simulink model "Driving_ACC_CACC_TL"  (R2016a)
settings: Solver=VariableStepAuto  StartTime=0.0  StopTime=10.0  RelTol=1e-3
undefined symbols (not defined in the file): ACCDelayDistance, ACCDelayVelocity, Area, ComfortAccelerationParameter, cR, cW, DeltaLeadVelocity, Epsilon, FuelConsumptionFactor, FuelConsumptionOffset, Mass, MaxBreakAcceleration, MaxLeadDistance, MaxSpeed, Power, StandstillDistance, StepTimeCoefficient, TimeGap
(part 1 of 2)
settings Model: Creator=Schlie  LastModifiedBy=Schlie

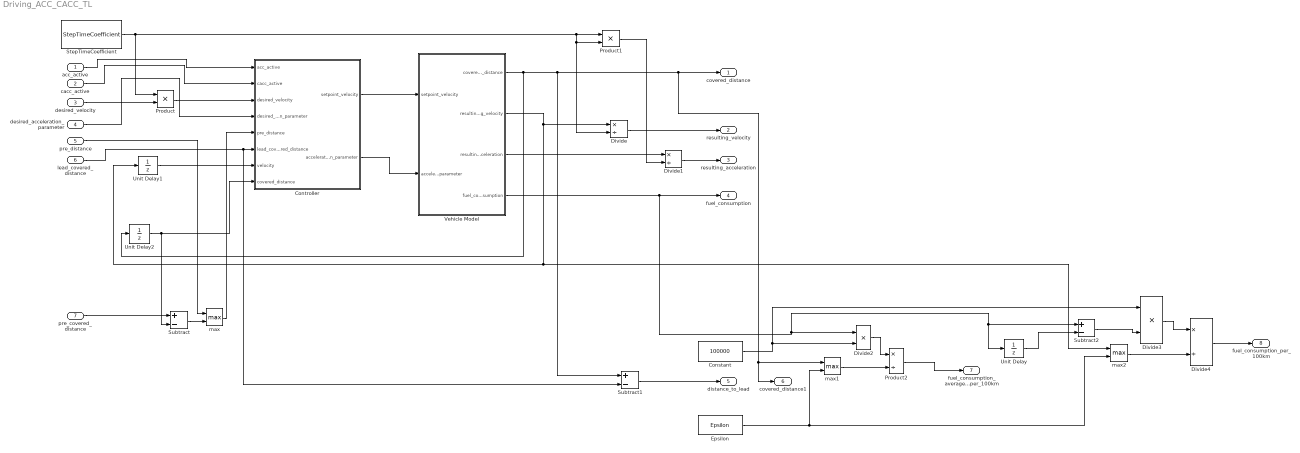
== system Driving_ACC_CACC_TL ==
  acc_active : Inport
      settings: DeleteFcn=if exist('delete_tlblock','file')==2,delete_tlblock(gcbh);end  OpenFcn=if exist('tl_open_blockdlg','file')==2,tl_open_blockdlg(gcbh);else,open_system(gcbh,'parameter');end
      settings: CopyFcn=|
      | if exist('tl_reset_reviewflag','file')==2
      |     tl_reset_reviewflag(gcbh);
      | end
      | if exist('tl_check_ports','file')
      |     tl_check_ports(gcbh);
      | end
      settings: NameChangeFcn=|
      | if exist('rename_tlblock','file')==2,rename_tlblock(gcbh);end
      | if exist('tl_check_ports','file'), tl_check_ports(gcbh); end
  cacc_active : Inport  Port=2
      settings: DeleteFcn=if exist('delete_tlblock','file')==2,delete_tlblock(gcbh);end  OpenFcn=if exist('tl_open_blockdlg','file')==2,tl_open_blockdlg(gcbh);else,open_system(gcbh,'parameter');end
      settings: CopyFcn=|
      | if exist('tl_reset_reviewflag','file')==2
      |     tl_reset_reviewflag(gcbh);
      | end
      | if exist('tl_check_ports','file')
      |     tl_check_ports(gcbh);
      | end
      settings: NameChangeFcn=|
      | if exist('rename_tlblock','file')==2,rename_tlblock(gcbh);end
      | if exist('tl_check_ports','file'), tl_check_ports(gcbh); end
  desired_velocity : Inport  Port=3
      settings: DeleteFcn=if exist('delete_tlblock','file')==2,delete_tlblock(gcbh);end  OpenFcn=if exist('tl_open_blockdlg','file')==2,tl_open_blockdlg(gcbh);else,open_system(gcbh,'parameter');end
      settings: CopyFcn=|
      | if exist('tl_reset_reviewflag','file')==2
      |     tl_reset_reviewflag(gcbh);
      | end
      | if exist('tl_check_ports','file')
      |     tl_check_ports(gcbh);
      | end
      settings: NameChangeFcn=|
      | if exist('rename_tlblock','file')==2,rename_tlblock(gcbh);end
      | if exist('tl_check_ports','file'), tl_check_ports(gcbh); end
  desired_acceleration_parameter : Inport  Port=4
      settings: DeleteFcn=if exist('delete_tlblock','file')==2,delete_tlblock(gcbh);end  OpenFcn=if exist('tl_open_blockdlg','file')==2,tl_open_blockdlg(gcbh);else,open_system(gcbh,'parameter');end
      settings: CopyFcn=|
      | if exist('tl_reset_reviewflag','file')==2
      |     tl_reset_reviewflag(gcbh);
      | end
      | if exist('tl_check_ports','file')
      |     tl_check_ports(gcbh);
      | end
      settings: NameChangeFcn=|
      | if exist('rename_tlblock','file')==2,rename_tlblock(gcbh);end
      | if exist('tl_check_ports','file'), tl_check_ports(gcbh); end
  pre_distance : Inport  Port=5
      settings: DeleteFcn=if exist('delete_tlblock','file')==2,delete_tlblock(gcbh);end  OpenFcn=if exist('tl_open_blockdlg','file')==2,tl_open_blockdlg(gcbh);else,open_system(gcbh,'parameter');end
      settings: CopyFcn=|
      | if exist('tl_reset_reviewflag','file')==2
      |     tl_reset_reviewflag(gcbh);
      | end
      | if exist('tl_check_ports','file')
      |     tl_check_ports(gcbh);
      | end
      settings: NameChangeFcn=|
      | if exist('rename_tlblock','file')==2,rename_tlblock(gcbh);end
      | if exist('tl_check_ports','file'), tl_check_ports(gcbh); end
  lead_covered_distance : Inport  Port=6
      settings: DeleteFcn=if exist('delete_tlblock','file')==2,delete_tlblock(gcbh);end  OpenFcn=if exist('tl_open_blockdlg','file')==2,tl_open_blockdlg(gcbh);else,open_system(gcbh,'parameter');end
      settings: CopyFcn=|
      | if exist('tl_reset_reviewflag','file')==2
      |     tl_reset_reviewflag(gcbh);
      | end
      | if exist('tl_check_ports','file')
      |     tl_check_ports(gcbh);
      | end
      settings: NameChangeFcn=|
      | if exist('rename_tlblock','file')==2,rename_tlblock(gcbh);end
      | if exist('tl_check_ports','file'), tl_check_ports(gcbh); end
  pre_covered_distance : Inport  Port=7
      settings: DeleteFcn=if exist('delete_tlblock','file')==2,delete_tlblock(gcbh);end  OpenFcn=if exist('tl_open_blockdlg','file')==2,tl_open_blockdlg(gcbh);else,open_system(gcbh,'parameter');end
      settings: CopyFcn=|
      | if exist('tl_reset_reviewflag','file')==2
      |     tl_reset_reviewflag(gcbh);
      | end
      | if exist('tl_check_ports','file')
      |     tl_check_ports(gcbh);
      | end
      settings: NameChangeFcn=|
      | if exist('rename_tlblock','file')==2,rename_tlblock(gcbh);end
      | if exist('tl_check_ports','file'), tl_check_ports(gcbh); end
  Constant : Constant  Value=100000
      settings: CopyFcn=if exist('tl_reset_reviewflag','file')==2,tl_reset_reviewflag(gcbh);end  DeleteFcn=if exist('delete_tlblock','file')==2,delete_tlblock(gcbh);end  NameChangeFcn=if exist('rename_tlblock','file')==2,rename_tlblock(gcbh);end  OpenFcn=if exist('tl_open_blockdlg','file')==2,tl_open_blockdlg(gcbh);else,open_system(gcbh,'parameter');end
  Controller : Subsystem
  Divide : Product  Inputs=*/
      settings: CopyFcn=if exist('tl_reset_reviewflag','file')==2,tl_reset_reviewflag(gcbh);end  DeleteFcn=if exist('delete_tlblock','file')==2,delete_tlblock(gcbh);end  NameChangeFcn=if exist('rename_tlblock','file')==2,rename_tlblock(gcbh);end  OpenFcn=if exist('tl_open_blockdlg','file')==2,tl_open_blockdlg(gcbh);else,open_system(gcbh,'parameter');end
  Divide1 : Product  Inputs=*/
      settings: CopyFcn=if exist('tl_reset_reviewflag','file')==2,tl_reset_reviewflag(gcbh);end  DeleteFcn=if exist('delete_tlblock','file')==2,delete_tlblock(gcbh);end  NameChangeFcn=if exist('rename_tlblock','file')==2,rename_tlblock(gcbh);end  OpenFcn=if exist('tl_open_blockdlg','file')==2,tl_open_blockdlg(gcbh);else,open_system(gcbh,'parameter');end
  Divide2 : Product  Inputs=**
      settings: CopyFcn=if exist('tl_reset_reviewflag','file')==2,tl_reset_reviewflag(gcbh);end  DeleteFcn=if exist('delete_tlblock','file')==2,delete_tlblock(gcbh);end  NameChangeFcn=if exist('rename_tlblock','file')==2,rename_tlblock(gcbh);end  OpenFcn=if exist('tl_open_blockdlg','file')==2,tl_open_blockdlg(gcbh);else,open_system(gcbh,'parameter');end
  Divide3 : Product  Inputs=**
      settings: CopyFcn=if exist('tl_reset_reviewflag','file')==2,tl_reset_reviewflag(gcbh);end  DeleteFcn=if exist('delete_tlblock','file')==2,delete_tlblock(gcbh);end  NameChangeFcn=if exist('rename_tlblock','file')==2,rename_tlblock(gcbh);end  OpenFcn=if exist('tl_open_blockdlg','file')==2,tl_open_blockdlg(gcbh);else,open_system(gcbh,'parameter');end
  Divide4 : Product  Inputs=*/
      settings: CopyFcn=if exist('tl_reset_reviewflag','file')==2,tl_reset_reviewflag(gcbh);end  DeleteFcn=if exist('delete_tlblock','file')==2,delete_tlblock(gcbh);end  NameChangeFcn=if exist('rename_tlblock','file')==2,rename_tlblock(gcbh);end  OpenFcn=if exist('tl_open_blockdlg','file')==2,tl_open_blockdlg(gcbh);else,open_system(gcbh,'parameter');end
  Epsilon : Constant  Value=Epsilon
      settings: CopyFcn=if exist('tl_reset_reviewflag','file')==2,tl_reset_reviewflag(gcbh);end  DeleteFcn=if exist('delete_tlblock','file')==2,delete_tlblock(gcbh);end  NameChangeFcn=if exist('rename_tlblock','file')==2,rename_tlblock(gcbh);end  OpenFcn=if exist('tl_open_blockdlg','file')==2,tl_open_blockdlg(gcbh);else,open_system(gcbh,'parameter');end
  Product : Product
      settings: CopyFcn=if exist('tl_reset_reviewflag','file')==2,tl_reset_reviewflag(gcbh);end  DeleteFcn=if exist('delete_tlblock','file')==2,delete_tlblock(gcbh);end  NameChangeFcn=if exist('rename_tlblock','file')==2,rename_tlblock(gcbh);end  OpenFcn=if exist('tl_open_blockdlg','file')==2,tl_open_blockdlg(gcbh);else,open_system(gcbh,'parameter');end
  Product1 : Product
      settings: CopyFcn=if exist('tl_reset_reviewflag','file')==2,tl_reset_reviewflag(gcbh);end  DeleteFcn=if exist('delete_tlblock','file')==2,delete_tlblock(gcbh);end  NameChangeFcn=if exist('rename_tlblock','file')==2,rename_tlblock(gcbh);end  OpenFcn=if exist('tl_open_blockdlg','file')==2,tl_open_blockdlg(gcbh);else,open_system(gcbh,'parameter');end
  Product2 : Product  Inputs=*/  RndMeth=Zero
      settings: CopyFcn=if exist('tl_reset_reviewflag') == 2, tl_reset_reviewflag(gcbh); end; if ~strcmp(get_param(gcbh, 'LinkStatus'), 'implicit') set_param(gcbh,'ReferenceBlock',''); end  DeleteFcn=if exist('delete_tlblock','file')==2,delete_tlblock(gcbh);end  NameChangeFcn=if exist('rename_tlblock','file')==2,rename_tlblock(gcbh);end  OpenFcn=if exist('tl_open_blockdlg','file')==2,tl_open_blockdlg(gcbh);else,open_system(gcbh,'parameter');end
  StepTimeCoefficient : Constant  Value=StepTimeCoefficient
      settings: CopyFcn=if exist('tl_reset_reviewflag','file')==2,tl_reset_reviewflag(gcbh);end  DeleteFcn=if exist('delete_tlblock','file')==2,delete_tlblock(gcbh);end  NameChangeFcn=if exist('rename_tlblock','file')==2,rename_tlblock(gcbh);end  OpenFcn=if exist('tl_open_blockdlg','file')==2,tl_open_blockdlg(gcbh);else,open_system(gcbh,'parameter');end
  Subtract : Sum  Inputs=+-
      settings: CopyFcn=if exist('tl_reset_reviewflag','file')==2,tl_reset_reviewflag(gcbh);end  DeleteFcn=if exist('delete_tlblock','file')==2,delete_tlblock(gcbh);end  NameChangeFcn=if exist('rename_tlblock','file')==2,rename_tlblock(gcbh);end  OpenFcn=if exist('tl_open_blockdlg','file')==2,tl_open_blockdlg(gcbh);else,open_system(gcbh,'parameter');end
  Subtract1 : Sum  Inputs=+-
      settings: CopyFcn=if exist('tl_reset_reviewflag','file')==2,tl_reset_reviewflag(gcbh);end  DeleteFcn=if exist('delete_tlblock','file')==2,delete_tlblock(gcbh);end  NameChangeFcn=if exist('rename_tlblock','file')==2,rename_tlblock(gcbh);end  OpenFcn=if exist('tl_open_blockdlg','file')==2,tl_open_blockdlg(gcbh);else,open_system(gcbh,'parameter');end
  Subtract2 : Sum  Inputs=+-
      settings: CopyFcn=if exist('tl_reset_reviewflag','file')==2,tl_reset_reviewflag(gcbh);end  DeleteFcn=if exist('delete_tlblock','file')==2,delete_tlblock(gcbh);end  NameChangeFcn=if exist('rename_tlblock','file')==2,rename_tlblock(gcbh);end  OpenFcn=if exist('tl_open_blockdlg','file')==2,tl_open_blockdlg(gcbh);else,open_system(gcbh,'parameter');end
  Unit Delay : UnitDelay  SampleTime=-1
      settings: CopyFcn=if exist('tl_reset_reviewflag','file')==2,tl_reset_reviewflag(gcbh);end  DeleteFcn=if exist('delete_tlblock','file')==2,delete_tlblock(gcbh);end  NameChangeFcn=if exist('rename_tlblock','file')==2,rename_tlblock(gcbh);end  OpenFcn=if exist('tl_open_blockdlg','file')==2,tl_open_blockdlg(gcbh);else,open_system(gcbh,'parameter');end
  Unit Delay1 : UnitDelay  SampleTime=-1
      settings: CopyFcn=if exist('tl_reset_reviewflag','file')==2,tl_reset_reviewflag(gcbh);end  DeleteFcn=if exist('delete_tlblock','file')==2,delete_tlblock(gcbh);end  NameChangeFcn=if exist('rename_tlblock','file')==2,rename_tlblock(gcbh);end  OpenFcn=if exist('tl_open_blockdlg','file')==2,tl_open_blockdlg(gcbh);else,open_system(gcbh,'parameter');end
  Unit Delay2 : UnitDelay  SampleTime=-1
      settings: CopyFcn=if exist('tl_reset_reviewflag','file')==2,tl_reset_reviewflag(gcbh);end  DeleteFcn=if exist('delete_tlblock','file')==2,delete_tlblock(gcbh);end  NameChangeFcn=if exist('rename_tlblock','file')==2,rename_tlblock(gcbh);end  OpenFcn=if exist('tl_open_blockdlg','file')==2,tl_open_blockdlg(gcbh);else,open_system(gcbh,'parameter');end
  Vehicle Model : Subsystem
  max : MinMax  Function=max  Inputs=2
      settings: CopyFcn=if exist('tl_reset_reviewflag','file')==2,tl_reset_reviewflag(gcbh);end  DeleteFcn=if exist('delete_tlblock','file')==2,delete_tlblock(gcbh);end  NameChangeFcn=if exist('rename_tlblock','file')==2,rename_tlblock(gcbh);end  OpenFcn=if exist('tl_open_blockdlg','file')==2,tl_open_blockdlg(gcbh);else,open_system(gcbh,'parameter');end
  max1 : MinMax  Function=max  Inputs=2
      settings: CopyFcn=if exist('tl_reset_reviewflag','file')==2,tl_reset_reviewflag(gcbh);end  DeleteFcn=if exist('delete_tlblock','file')==2,delete_tlblock(gcbh);end  NameChangeFcn=if exist('rename_tlblock','file')==2,rename_tlblock(gcbh);end  OpenFcn=if exist('tl_open_blockdlg','file')==2,tl_open_blockdlg(gcbh);else,open_system(gcbh,'parameter');end
  max2 : MinMax  Function=max  Inputs=2
      settings: CopyFcn=if exist('tl_reset_reviewflag','file')==2,tl_reset_reviewflag(gcbh);end  DeleteFcn=if exist('delete_tlblock','file')==2,delete_tlblock(gcbh);end  NameChangeFcn=if exist('rename_tlblock','file')==2,rename_tlblock(gcbh);end  OpenFcn=if exist('tl_open_blockdlg','file')==2,tl_open_blockdlg(gcbh);else,open_system(gcbh,'parameter');end
  covered_distance : Outport
      settings: DeleteFcn=if exist('delete_tlblock','file')==2,delete_tlblock(gcbh);end  OpenFcn=if exist('tl_open_blockdlg','file')==2,tl_open_blockdlg(gcbh);else,open_system(gcbh,'parameter');end
      settings: CopyFcn=|
      | if exist('tl_reset_reviewflag','file')==2
      |     tl_reset_reviewflag(gcbh);
      | end
      | if exist('tl_check_ports','file')
      |     tl_check_ports(gcbh);
      | end
      settings: NameChangeFcn=|
      | if exist('rename_tlblock','file')==2,rename_tlblock(gcbh);end
      | if exist('tl_check_ports','file'), tl_check_ports(gcbh); end
  resulting_velocity : Outport  Port=2
      settings: DeleteFcn=if exist('delete_tlblock','file')==2,delete_tlblock(gcbh);end  OpenFcn=if exist('tl_open_blockdlg','file')==2,tl_open_blockdlg(gcbh);else,open_system(gcbh,'parameter');end
      settings: CopyFcn=|
      | if exist('tl_reset_reviewflag','file')==2
      |     tl_reset_reviewflag(gcbh);
      | end
      | if exist('tl_check_ports','file')
      |     tl_check_ports(gcbh);
      | end
      settings: NameChangeFcn=|
      | if exist('rename_tlblock','file')==2,rename_tlblock(gcbh);end
      | if exist('tl_check_ports','file'), tl_check_ports(gcbh); end
  resulting_acceleration : Outport  Port=3
      settings: DeleteFcn=if exist('delete_tlblock','file')==2,delete_tlblock(gcbh);end  OpenFcn=if exist('tl_open_blockdlg','file')==2,tl_open_blockdlg(gcbh);else,open_system(gcbh,'parameter');end
      settings: CopyFcn=|
      | if exist('tl_reset_reviewflag','file')==2
      |     tl_reset_reviewflag(gcbh);
      | end
      | if exist('tl_check_ports','file')
      |     tl_check_ports(gcbh);
      | end
      settings: NameChangeFcn=|
      | if exist('rename_tlblock','file')==2,rename_tlblock(gcbh);end
      | if exist('tl_check_ports','file'), tl_check_ports(gcbh); end
  fuel_consumption : Outport  Port=4
      settings: DeleteFcn=if exist('delete_tlblock','file')==2,delete_tlblock(gcbh);end  OpenFcn=if exist('tl_open_blockdlg','file')==2,tl_open_blockdlg(gcbh);else,open_system(gcbh,'parameter');end
      settings: CopyFcn=|
      | if exist('tl_reset_reviewflag','file')==2
      |     tl_reset_reviewflag(gcbh);
      | end
      | if exist('tl_check_ports','file')
      |     tl_check_ports(gcbh);
      | end
      settings: NameChangeFcn=|
      | if exist('rename_tlblock','file')==2,rename_tlblock(gcbh);end
      | if exist('tl_check_ports','file'), tl_check_ports(gcbh); end
  distance_to_lead : Outport  Port=5
      settings: DeleteFcn=if exist('delete_tlblock','file')==2,delete_tlblock(gcbh);end  OpenFcn=if exist('tl_open_blockdlg','file')==2,tl_open_blockdlg(gcbh);else,open_system(gcbh,'parameter');end
      settings: CopyFcn=|
      | if exist('tl_reset_reviewflag','file')==2
      |     tl_reset_reviewflag(gcbh);
      | end
      | if exist('tl_check_ports','file')
      |     tl_check_ports(gcbh);
      | end
      settings: NameChangeFcn=|
      | if exist('rename_tlblock','file')==2,rename_tlblock(gcbh);end
      | if exist('tl_check_ports','file'), tl_check_ports(gcbh); end
  covered_distance1 : Outport  Port=6
      settings: DeleteFcn=if exist('delete_tlblock','file')==2,delete_tlblock(gcbh);end  OpenFcn=if exist('tl_open_blockdlg','file')==2,tl_open_blockdlg(gcbh);else,open_system(gcbh,'parameter');end
      settings: CopyFcn=|
      | if exist('tl_reset_reviewflag','file')==2
      |     tl_reset_reviewflag(gcbh);
      | end
      | if exist('tl_check_ports','file')
      |     tl_check_ports(gcbh);
      | end
      settings: NameChangeFcn=|
      | if exist('rename_tlblock','file')==2,rename_tlblock(gcbh);end
      | if exist('tl_check_ports','file'), tl_check_ports(gcbh); end
  fuel_consumption_average_per_100km : Outport  Port=7
      settings: DeleteFcn=if exist('delete_tlblock','file')==2,delete_tlblock(gcbh);end  OpenFcn=if exist('tl_open_blockdlg','file')==2,tl_open_blockdlg(gcbh);else,open_system(gcbh,'parameter');end
      settings: CopyFcn=|
      | if exist('tl_reset_reviewflag','file')==2
      |     tl_reset_reviewflag(gcbh);
      | end
      | if exist('tl_check_ports','file')
      |     tl_check_ports(gcbh);
      | end
      settings: NameChangeFcn=|
      | if exist('rename_tlblock','file')==2,rename_tlblock(gcbh);end
      | if exist('tl_check_ports','file'), tl_check_ports(gcbh); end
  fuel_consumption_per_100km : Outport  Port=8
      settings: DeleteFcn=if exist('delete_tlblock','file')==2,delete_tlblock(gcbh);end  OpenFcn=if exist('tl_open_blockdlg','file')==2,tl_open_blockdlg(gcbh);else,open_system(gcbh,'parameter');end
      settings: CopyFcn=|
      | if exist('tl_reset_reviewflag','file')==2
      |     tl_reset_reviewflag(gcbh);
      | end
      | if exist('tl_check_ports','file')
      |     tl_check_ports(gcbh);
      | end
      settings: NameChangeFcn=|
      | if exist('rename_tlblock','file')==2,rename_tlblock(gcbh);end
      | if exist('tl_check_ports','file'), tl_check_ports(gcbh); end
  wires:
  lead_covered_distance/1 -> Subtract1/2, Controller/6(lead_covered_distance)
  Vehicle Model/2(resulting_velocity) -> Divide/1, Unit Delay1/1, max2/1
  acc_active/1 -> Controller/1(acc_active)
  desired_velocity/1 -> Product/2
  StepTimeCoefficient/1 -> Product1/1, Product1/2, Divide/2, Product/1
  Divide1/1 -> resulting_acceleration/1
  Vehicle Model/1(covered_distance) -> Unit Delay2/1, Subtract1/1, covered_distance/1, covered_distance1/1, max1/1
  Divide/1 -> resulting_velocity/1
  cacc_active/1 -> Controller/2(cacc_active)
  Product/1 -> Controller/3(desired_velocity)
  pre_distance/1 -> max/1
  Vehicle Model/3(resulting_acceleration) -> Divide1/1
  Controller/2(acceleration_parameter) -> Vehicle Model/2(acceleration_parameter)
  Constant/1 -> Divide3/1, Divide2/2
  Controller/1(setpoint_velocity) -> Vehicle Model/1(setpoint_velocity)
  Subtract2/1 -> Divide3/2
  max1/1 -> Product2/2
  Subtract/1 -> max/2
  Unit Delay/1 -> Subtract2/2
  pre_covered_distance/1 -> Subtract/1
  Subtract1/1 -> distance_to_lead/1
  Vehicle Model/4(fuel_consumption) -> fuel_consumption/1, Unit Delay/1, Subtract2/1, Divide2/1
  max2/1 -> Divide4/2
  desired_acceleration_parameter/1 -> Controller/4(desired_acceleration_parameter)
  Epsilon/1 -> max2/2, max1/2
  max/1 -> Controller/5(pre_distance)
  Product1/1 -> Divide1/2
  Unit Delay1/1 -> Controller/7(velocity)
  Unit Delay2/1 -> Controller/8(covered_distance), Subtract/2
  Divide2/1 -> Product2/1
  Product2/1 -> fuel_consumption_average_per_100km/1
  Divide3/1 -> Divide4/1
  Divide4/1 -> fuel_consumption_per_100km/1

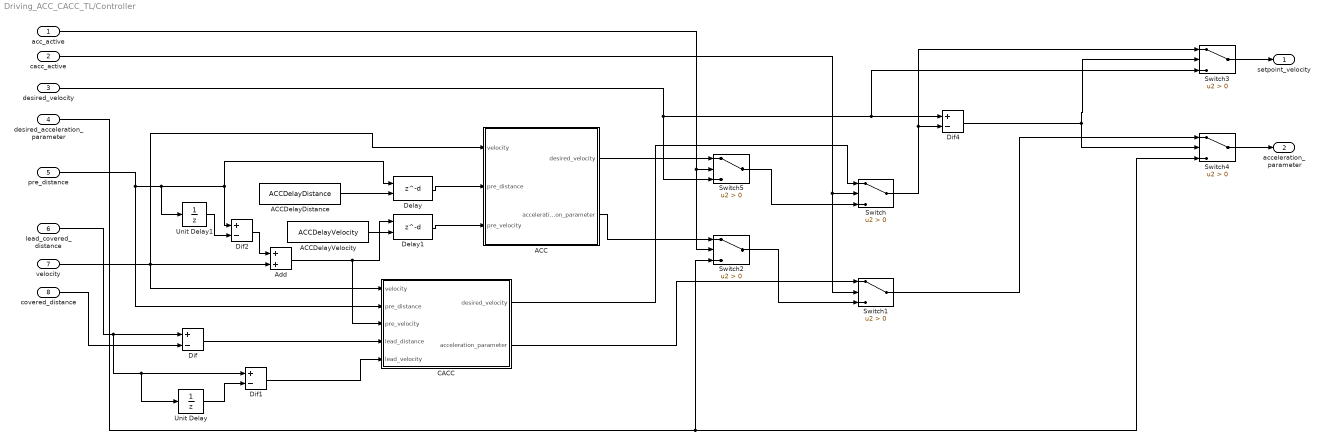
== system Driving_ACC_CACC_TL/Controller ==
  acc_active : Inport
      settings: CopyFcn=if exist('tl_reset_reviewflag','file')==2,tl_reset_reviewflag(gcbh);end  DeleteFcn=if exist('delete_tlblock','file')==2,delete_tlblock(gcbh);end  NameChangeFcn=if exist('rename_tlblock','file')==2,rename_tlblock(gcbh);end  OpenFcn=if exist('tl_open_blockdlg','file')==2,tl_open_blockdlg(gcbh);else,open_system(gcbh,'parameter');end
  cacc_active : Inport  Port=2
      settings: CopyFcn=if exist('tl_reset_reviewflag','file')==2,tl_reset_reviewflag(gcbh);end  DeleteFcn=if exist('delete_tlblock','file')==2,delete_tlblock(gcbh);end  NameChangeFcn=if exist('rename_tlblock','file')==2,rename_tlblock(gcbh);end  OpenFcn=if exist('tl_open_blockdlg','file')==2,tl_open_blockdlg(gcbh);else,open_system(gcbh,'parameter');end
  desired_velocity : Inport  Port=3
      settings: CopyFcn=if exist('tl_reset_reviewflag','file')==2,tl_reset_reviewflag(gcbh);end  DeleteFcn=if exist('delete_tlblock','file')==2,delete_tlblock(gcbh);end  NameChangeFcn=if exist('rename_tlblock','file')==2,rename_tlblock(gcbh);end  OpenFcn=if exist('tl_open_blockdlg','file')==2,tl_open_blockdlg(gcbh);else,open_system(gcbh,'parameter');end
  desired_acceleration_parameter : Inport  Port=4
      settings: CopyFcn=if exist('tl_reset_reviewflag','file')==2,tl_reset_reviewflag(gcbh);end  DeleteFcn=if exist('delete_tlblock','file')==2,delete_tlblock(gcbh);end  NameChangeFcn=if exist('rename_tlblock','file')==2,rename_tlblock(gcbh);end  OpenFcn=if exist('tl_open_blockdlg','file')==2,tl_open_blockdlg(gcbh);else,open_system(gcbh,'parameter');end
  pre_distance : Inport  Port=5
      settings: CopyFcn=if exist('tl_reset_reviewflag','file')==2,tl_reset_reviewflag(gcbh);end  DeleteFcn=if exist('delete_tlblock','file')==2,delete_tlblock(gcbh);end  NameChangeFcn=if exist('rename_tlblock','file')==2,rename_tlblock(gcbh);end  OpenFcn=if exist('tl_open_blockdlg','file')==2,tl_open_blockdlg(gcbh);else,open_system(gcbh,'parameter');end
  lead_covered_distance : Inport  Port=6
      settings: CopyFcn=if exist('tl_reset_reviewflag','file')==2,tl_reset_reviewflag(gcbh);end  DeleteFcn=if exist('delete_tlblock','file')==2,delete_tlblock(gcbh);end  NameChangeFcn=if exist('rename_tlblock','file')==2,rename_tlblock(gcbh);end  OpenFcn=if exist('tl_open_blockdlg','file')==2,tl_open_blockdlg(gcbh);else,open_system(gcbh,'parameter');end
  velocity : Inport  Port=7
      settings: CopyFcn=if exist('tl_reset_reviewflag','file')==2,tl_reset_reviewflag(gcbh);end  DeleteFcn=if exist('delete_tlblock','file')==2,delete_tlblock(gcbh);end  NameChangeFcn=if exist('rename_tlblock','file')==2,rename_tlblock(gcbh);end  OpenFcn=if exist('tl_open_blockdlg','file')==2,tl_open_blockdlg(gcbh);else,open_system(gcbh,'parameter');end
  covered_distance : Inport  Port=8
      settings: CopyFcn=if exist('tl_reset_reviewflag','file')==2,tl_reset_reviewflag(gcbh);end  DeleteFcn=if exist('delete_tlblock','file')==2,delete_tlblock(gcbh);end  NameChangeFcn=if exist('rename_tlblock','file')==2,rename_tlblock(gcbh);end  OpenFcn=if exist('tl_open_blockdlg','file')==2,tl_open_blockdlg(gcbh);else,open_system(gcbh,'parameter');end
  ACC : Subsystem
  ACCDelayDistance : Constant  Value=ACCDelayDistance
      settings: CopyFcn=if exist('tl_reset_reviewflag','file')==2,tl_reset_reviewflag(gcbh);end  DeleteFcn=if exist('delete_tlblock','file')==2,delete_tlblock(gcbh);end  NameChangeFcn=if exist('rename_tlblock','file')==2,rename_tlblock(gcbh);end  OpenFcn=if exist('tl_open_blockdlg','file')==2,tl_open_blockdlg(gcbh);else,open_system(gcbh,'parameter');end
  ACCDelayVelocity : Constant  Value=ACCDelayVelocity
      settings: CopyFcn=if exist('tl_reset_reviewflag','file')==2,tl_reset_reviewflag(gcbh);end  DeleteFcn=if exist('delete_tlblock','file')==2,delete_tlblock(gcbh);end  NameChangeFcn=if exist('rename_tlblock','file')==2,rename_tlblock(gcbh);end  OpenFcn=if exist('tl_open_blockdlg','file')==2,tl_open_blockdlg(gcbh);else,open_system(gcbh,'parameter');end
  Add : Sum
      settings: CopyFcn=if exist('tl_reset_reviewflag','file')==2,tl_reset_reviewflag(gcbh);end  DeleteFcn=if exist('delete_tlblock','file')==2,delete_tlblock(gcbh);end  NameChangeFcn=if exist('rename_tlblock','file')==2,rename_tlblock(gcbh);end  OpenFcn=if exist('tl_open_blockdlg','file')==2,tl_open_blockdlg(gcbh);else,open_system(gcbh,'parameter');end
  CACC : Subsystem
  Delay : Delay  DelayLengthSource=Input port  DelayLength=ACCDelayDistance
      settings: CopyFcn=if exist('tl_reset_reviewflag','file')==2,tl_reset_reviewflag(gcbh);end  DeleteFcn=if exist('delete_tlblock','file')==2,delete_tlblock(gcbh);end  NameChangeFcn=if exist('rename_tlblock','file')==2,rename_tlblock(gcbh);end  OpenFcn=if exist('tl_open_blockdlg','file')==2,tl_open_blockdlg(gcbh);else,open_system(gcbh,'parameter');end  InputPortMap=u0,p1
  Delay1 : Delay  DelayLengthSource=Input port  DelayLength=ACCDelayVelocity
      settings: CopyFcn=if exist('tl_reset_reviewflag','file')==2,tl_reset_reviewflag(gcbh);end  DeleteFcn=if exist('delete_tlblock','file')==2,delete_tlblock(gcbh);end  NameChangeFcn=if exist('rename_tlblock','file')==2,rename_tlblock(gcbh);end  OpenFcn=if exist('tl_open_blockdlg','file')==2,tl_open_blockdlg(gcbh);else,open_system(gcbh,'parameter');end  InputPortMap=u0,p1
  Dif{,1..2,4} (4 alike) : Sum  Inputs=+-
      settings: CopyFcn=if exist('tl_reset_reviewflag','file')==2,tl_reset_reviewflag(gcbh);end  DeleteFcn=if exist('delete_tlblock','file')==2,delete_tlblock(gcbh);end  NameChangeFcn=if exist('rename_tlblock','file')==2,rename_tlblock(gcbh);end  OpenFcn=if exist('tl_open_blockdlg','file')==2,tl_open_blockdlg(gcbh);else,open_system(gcbh,'parameter');end
  Switch{,1..5} (6 alike) : Switch  Criteria=u2 > Threshold
      settings: CopyFcn=if exist('tl_reset_reviewflag','file')==2,tl_reset_reviewflag(gcbh);end  DeleteFcn=if exist('delete_tlblock','file')==2,delete_tlblock(gcbh);end  NameChangeFcn=if exist('rename_tlblock','file')==2,rename_tlblock(gcbh);end  OpenFcn=if exist('tl_open_blockdlg','file')==2,tl_open_blockdlg(gcbh);else,open_system(gcbh,'parameter');end
  Unit Delay : UnitDelay  SampleTime=-1
      settings: CopyFcn=if exist('tl_reset_reviewflag','file')==2,tl_reset_reviewflag(gcbh);end  DeleteFcn=if exist('delete_tlblock','file')==2,delete_tlblock(gcbh);end  NameChangeFcn=if exist('rename_tlblock','file')==2,rename_tlblock(gcbh);end  OpenFcn=if exist('tl_open_blockdlg','file')==2,tl_open_blockdlg(gcbh);else,open_system(gcbh,'parameter');end
  Unit Delay1 : UnitDelay  SampleTime=-1
      settings: CopyFcn=if exist('tl_reset_reviewflag','file')==2,tl_reset_reviewflag(gcbh);end  DeleteFcn=if exist('delete_tlblock','file')==2,delete_tlblock(gcbh);end  NameChangeFcn=if exist('rename_tlblock','file')==2,rename_tlblock(gcbh);end  OpenFcn=if exist('tl_open_blockdlg','file')==2,tl_open_blockdlg(gcbh);else,open_system(gcbh,'parameter');end
  setpoint_velocity : Outport
      settings: CopyFcn=if exist('tl_reset_reviewflag','file')==2,tl_reset_reviewflag(gcbh);end  DeleteFcn=if exist('delete_tlblock','file')==2,delete_tlblock(gcbh);end  NameChangeFcn=if exist('rename_tlblock','file')==2,rename_tlblock(gcbh);end  OpenFcn=if exist('tl_open_blockdlg','file')==2,tl_open_blockdlg(gcbh);else,open_system(gcbh,'parameter');end
  acceleration_parameter : Outport  Port=2
      settings: CopyFcn=if exist('tl_reset_reviewflag','file')==2,tl_reset_reviewflag(gcbh);end  DeleteFcn=if exist('delete_tlblock','file')==2,delete_tlblock(gcbh);end  NameChangeFcn=if exist('rename_tlblock','file')==2,rename_tlblock(gcbh);end  OpenFcn=if exist('tl_open_blockdlg','file')==2,tl_open_blockdlg(gcbh);else,open_system(gcbh,'parameter');end
  wires:
  velocity/1 -> ACC/1(velocity), Add/2, CACC/1(velocity)
  Add/1 -> Delay1/1, CACC/3(pre_velocity)
  lead_covered_distance/1 -> Unit Delay/1, Dif1/1, Dif/1
  covered_distance/1 -> Dif/2
  Dif/1 -> CACC/4(lead_distance)
  Dif1/1 -> CACC/5(lead_velocity)
  Switch3/1 -> setpoint_velocity/1
  desired_velocity/1 -> Switch5/3, Switch3/3, Dif4/1
  Switch4/1 -> acceleration_parameter/1
  Dif2/1 -> Add/1
  Unit Delay/1 -> Dif1/2
  pre_distance/1 -> CACC/2(pre_distance), Unit Delay1/1, Delay/1, Dif2/1
  desired_acceleration_parameter/1 -> Switch2/3, Switch4/3
  Delay/1 -> ACC/2(pre_distance)
  Delay1/1 -> ACC/3(pre_velocity)
  Switch/1 -> Switch3/1, Dif4/2
  Dif4/1 -> Switch3/2, Switch4/2
  Switch1/1 -> Switch4/1
  cacc_active/1 -> Switch1/2, Switch/2
  CACC/1(desired_velocity) -> Switch/1
  CACC/2(acceleration_parameter) -> Switch1/1
  Switch2/1 -> Switch1/3
  Switch5/1 -> Switch/3
  acc_active/1 -> Switch2/2, Switch5/2
  ACC/2(acceleration_parameter) -> Switch2/1
  ACC/1(desired_velocity) -> Switch5/1
  ACCDelayDistance/1 -> Delay/2
  ACCDelayVelocity/1 -> Delay1/2
  Unit Delay1/1 -> Dif2/2

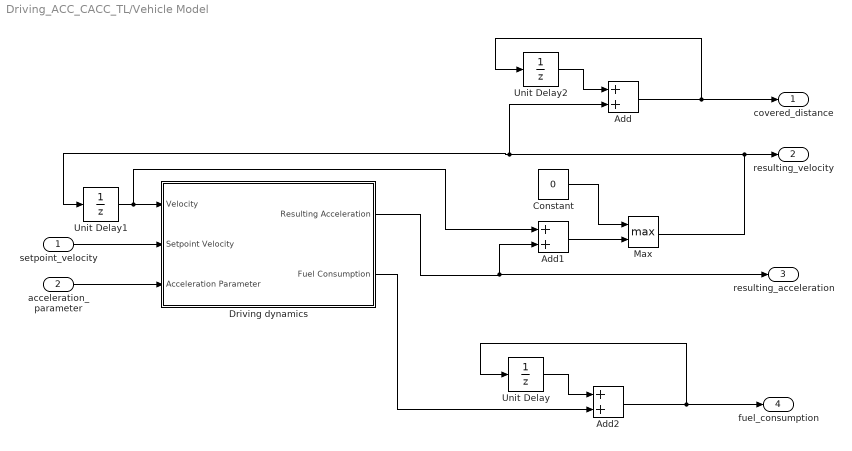
== system Driving_ACC_CACC_TL/Vehicle Model ==
  setpoint_velocity : Inport
  acceleration_parameter : Inport  Port=2
  Add : Sum
      settings: CopyFcn=if exist('tl_reset_reviewflag','file')==2,tl_reset_reviewflag(gcbh);end  DeleteFcn=if exist('delete_tlblock','file')==2,delete_tlblock(gcbh);end  NameChangeFcn=if exist('rename_tlblock','file')==2,rename_tlblock(gcbh);end  OpenFcn=if exist('tl_open_blockdlg','file')==2,tl_open_blockdlg(gcbh);else,open_system(gcbh,'parameter');end
  Add1 : Sum
      settings: CopyFcn=if exist('tl_reset_reviewflag','file')==2,tl_reset_reviewflag(gcbh);end  DeleteFcn=if exist('delete_tlblock','file')==2,delete_tlblock(gcbh);end  NameChangeFcn=if exist('rename_tlblock','file')==2,rename_tlblock(gcbh);end  OpenFcn=if exist('tl_open_blockdlg','file')==2,tl_open_blockdlg(gcbh);else,open_system(gcbh,'parameter');end
  Add2 : Sum
      settings: CopyFcn=if exist('tl_reset_reviewflag','file')==2,tl_reset_reviewflag(gcbh);end  DeleteFcn=if exist('delete_tlblock','file')==2,delete_tlblock(gcbh);end  NameChangeFcn=if exist('rename_tlblock','file')==2,rename_tlblock(gcbh);end  OpenFcn=if exist('tl_open_blockdlg','file')==2,tl_open_blockdlg(gcbh);else,open_system(gcbh,'parameter');end
  Constant : Constant  Value=0
      settings: CopyFcn=if exist('tl_reset_reviewflag','file')==2,tl_reset_reviewflag(gcbh);end  DeleteFcn=if exist('delete_tlblock','file')==2,delete_tlblock(gcbh);end  NameChangeFcn=if exist('rename_tlblock','file')==2,rename_tlblock(gcbh);end  OpenFcn=if exist('tl_open_blockdlg','file')==2,tl_open_blockdlg(gcbh);else,open_system(gcbh,'parameter');end
  Driving dynamics : Subsystem
  Max : MinMax  Function=max  Inputs=2
      settings: CopyFcn=if exist('tl_reset_reviewflag','file')==2,tl_reset_reviewflag(gcbh);end  DeleteFcn=if exist('delete_tlblock','file')==2,delete_tlblock(gcbh);end  NameChangeFcn=if exist('rename_tlblock','file')==2,rename_tlblock(gcbh);end  OpenFcn=if exist('tl_open_blockdlg','file')==2,tl_open_blockdlg(gcbh);else,open_system(gcbh,'parameter');end
  Unit Delay : UnitDelay  SampleTime=-1
      settings: CopyFcn=if exist('tl_reset_reviewflag','file')==2,tl_reset_reviewflag(gcbh);end  DeleteFcn=if exist('delete_tlblock','file')==2,delete_tlblock(gcbh);end  NameChangeFcn=if exist('rename_tlblock','file')==2,rename_tlblock(gcbh);end  OpenFcn=if exist('tl_open_blockdlg','file')==2,tl_open_blockdlg(gcbh);else,open_system(gcbh,'parameter');end
  Unit Delay1 : UnitDelay  SampleTime=-1
      settings: CopyFcn=if exist('tl_reset_reviewflag','file')==2,tl_reset_reviewflag(gcbh);end  DeleteFcn=if exist('delete_tlblock','file')==2,delete_tlblock(gcbh);end  NameChangeFcn=if exist('rename_tlblock','file')==2,rename_tlblock(gcbh);end  OpenFcn=if exist('tl_open_blockdlg','file')==2,tl_open_blockdlg(gcbh);else,open_system(gcbh,'parameter');end
  Unit Delay2 : UnitDelay  SampleTime=-1
      settings: CopyFcn=if exist('tl_reset_reviewflag','file')==2,tl_reset_reviewflag(gcbh);end  DeleteFcn=if exist('delete_tlblock','file')==2,delete_tlblock(gcbh);end  NameChangeFcn=if exist('rename_tlblock','file')==2,rename_tlblock(gcbh);end  OpenFcn=if exist('tl_open_blockdlg','file')==2,tl_open_blockdlg(gcbh);else,open_system(gcbh,'parameter');end
  covered_distance : Outport
  resulting_velocity : Outport  Port=2
  resulting_acceleration : Outport  Port=3
  fuel_consumption : Outport  Port=4
  wires:
  Add/1 -> Unit Delay2/1, covered_distance/1
  Max/1 -> Unit Delay1/1, Add/2, resulting_velocity/1
  setpoint_velocity/1 -> Driving dynamics/2(Setpoint Velocity)
  acceleration_parameter/1 -> Driving dynamics/3(Acceleration Parameter)
  Unit Delay1/1 -> Add1/1, Driving dynamics/1(Velocity)
  Unit Delay2/1 -> Add/1
  Driving dynamics/1(Resulting Acceleration) -> Add1/2, resulting_acceleration/1
  Add1/1 -> Max/2
  Constant/1 -> Max/1
  Add2/1 -> Unit Delay/1, fuel_consumption/1
  Driving dynamics/2(Fuel Consumption) -> Add2/2
  Unit Delay/1 -> Add2/1

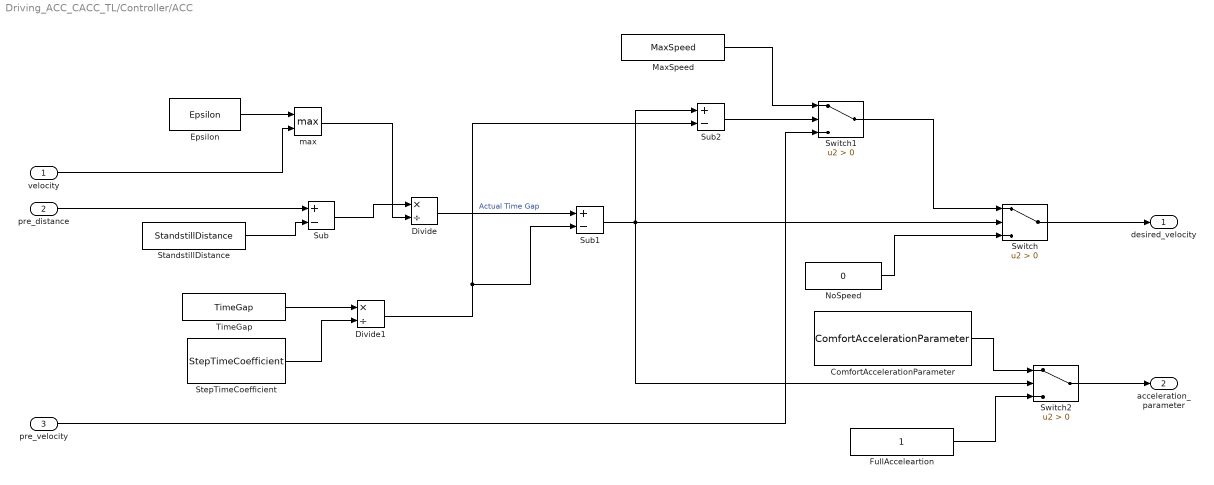
== system Driving_ACC_CACC_TL/Controller/ACC ==
  velocity : Inport
  pre_distance : Inport  Port=2
  pre_velocity : Inport  Port=3
  ComfortAccelerationParameter : Constant  Value=ComfortAccelerationParameter
      settings: CopyFcn=if exist('tl_reset_reviewflag','file')==2,tl_reset_reviewflag(gcbh);end  DeleteFcn=if exist('delete_tlblock','file')==2,delete_tlblock(gcbh);end  NameChangeFcn=if exist('rename_tlblock','file')==2,rename_tlblock(gcbh);end  OpenFcn=if exist('tl_open_blockdlg','file')==2,tl_open_blockdlg(gcbh);else,open_system(gcbh,'parameter');end
  Divide : Product  Inputs=*/
      settings: CopyFcn=if exist('tl_reset_reviewflag','file')==2,tl_reset_reviewflag(gcbh);end  DeleteFcn=if exist('delete_tlblock','file')==2,delete_tlblock(gcbh);end  NameChangeFcn=if exist('rename_tlblock','file')==2,rename_tlblock(gcbh);end  OpenFcn=if exist('tl_open_blockdlg','file')==2,tl_open_blockdlg(gcbh);else,open_system(gcbh,'parameter');end
  Divide1 : Product  Inputs=*/
      settings: CopyFcn=if exist('tl_reset_reviewflag','file')==2,tl_reset_reviewflag(gcbh);end  DeleteFcn=if exist('delete_tlblock','file')==2,delete_tlblock(gcbh);end  NameChangeFcn=if exist('rename_tlblock','file')==2,rename_tlblock(gcbh);end  OpenFcn=if exist('tl_open_blockdlg','file')==2,tl_open_blockdlg(gcbh);else,open_system(gcbh,'parameter');end
  Epsilon : Constant  Value=Epsilon
      settings: CopyFcn=if exist('tl_reset_reviewflag','file')==2,tl_reset_reviewflag(gcbh);end  DeleteFcn=if exist('delete_tlblock','file')==2,delete_tlblock(gcbh);end  NameChangeFcn=if exist('rename_tlblock','file')==2,rename_tlblock(gcbh);end  OpenFcn=if exist('tl_open_blockdlg','file')==2,tl_open_blockdlg(gcbh);else,open_system(gcbh,'parameter');end
  FullAcceleartion : Constant
      settings: CopyFcn=if exist('tl_reset_reviewflag','file')==2,tl_reset_reviewflag(gcbh);end  DeleteFcn=if exist('delete_tlblock','file')==2,delete_tlblock(gcbh);end  NameChangeFcn=if exist('rename_tlblock','file')==2,rename_tlblock(gcbh);end  OpenFcn=if exist('tl_open_blockdlg','file')==2,tl_open_blockdlg(gcbh);else,open_system(gcbh,'parameter');end
  MaxSpeed : Constant  Value=MaxSpeed
      settings: CopyFcn=if exist('tl_reset_reviewflag','file')==2,tl_reset_reviewflag(gcbh);end  DeleteFcn=if exist('delete_tlblock','file')==2,delete_tlblock(gcbh);end  NameChangeFcn=if exist('rename_tlblock','file')==2,rename_tlblock(gcbh);end  OpenFcn=if exist('tl_open_blockdlg','file')==2,tl_open_blockdlg(gcbh);else,open_system(gcbh,'parameter');end
  NoSpeed : Constant  Value=0
      settings: CopyFcn=if exist('tl_reset_reviewflag','file')==2,tl_reset_reviewflag(gcbh);end  DeleteFcn=if exist('delete_tlblock','file')==2,delete_tlblock(gcbh);end  NameChangeFcn=if exist('rename_tlblock','file')==2,rename_tlblock(gcbh);end  OpenFcn=if exist('tl_open_blockdlg','file')==2,tl_open_blockdlg(gcbh);else,open_system(gcbh,'parameter');end
  StandstillDistance : Constant  Value=StandstillDistance
      settings: CopyFcn=if exist('tl_reset_reviewflag','file')==2,tl_reset_reviewflag(gcbh);end  DeleteFcn=if exist('delete_tlblock','file')==2,delete_tlblock(gcbh);end  NameChangeFcn=if exist('rename_tlblock','file')==2,rename_tlblock(gcbh);end  OpenFcn=if exist('tl_open_blockdlg','file')==2,tl_open_blockdlg(gcbh);else,open_system(gcbh,'parameter');end
  StepTimeCoefficient : Constant  Value=StepTimeCoefficient
      settings: CopyFcn=if exist('tl_reset_reviewflag','file')==2,tl_reset_reviewflag(gcbh);end  DeleteFcn=if exist('delete_tlblock','file')==2,delete_tlblock(gcbh);end  NameChangeFcn=if exist('rename_tlblock','file')==2,rename_tlblock(gcbh);end  OpenFcn=if exist('tl_open_blockdlg','file')==2,tl_open_blockdlg(gcbh);else,open_system(gcbh,'parameter');end
  Sub : Sum  Inputs=+-
      settings: CopyFcn=if exist('tl_reset_reviewflag','file')==2,tl_reset_reviewflag(gcbh);end  DeleteFcn=if exist('delete_tlblock','file')==2,delete_tlblock(gcbh);end  NameChangeFcn=if exist('rename_tlblock','file')==2,rename_tlblock(gcbh);end  OpenFcn=if exist('tl_open_blockdlg','file')==2,tl_open_blockdlg(gcbh);else,open_system(gcbh,'parameter');end
  Sub1 : Sum  Inputs=+-
      settings: CopyFcn=if exist('tl_reset_reviewflag','file')==2,tl_reset_reviewflag(gcbh);end  DeleteFcn=if exist('delete_tlblock','file')==2,delete_tlblock(gcbh);end  NameChangeFcn=if exist('rename_tlblock','file')==2,rename_tlblock(gcbh);end  OpenFcn=if exist('tl_open_blockdlg','file')==2,tl_open_blockdlg(gcbh);else,open_system(gcbh,'parameter');end
  Sub2 : Sum  Inputs=+-
      settings: CopyFcn=if exist('tl_reset_reviewflag','file')==2,tl_reset_reviewflag(gcbh);end  DeleteFcn=if exist('delete_tlblock','file')==2,delete_tlblock(gcbh);end  NameChangeFcn=if exist('rename_tlblock','file')==2,rename_tlblock(gcbh);end  OpenFcn=if exist('tl_open_blockdlg','file')==2,tl_open_blockdlg(gcbh);else,open_system(gcbh,'parameter');end
  Switch : Switch  Criteria=u2 > Threshold
      settings: CopyFcn=if exist('tl_reset_reviewflag','file')==2,tl_reset_reviewflag(gcbh);end  DeleteFcn=if exist('delete_tlblock','file')==2,delete_tlblock(gcbh);end  NameChangeFcn=if exist('rename_tlblock','file')==2,rename_tlblock(gcbh);end  OpenFcn=if exist('tl_open_blockdlg','file')==2,tl_open_blockdlg(gcbh);else,open_system(gcbh,'parameter');end
  Switch1 : Switch  Criteria=u2 > Threshold
      settings: CopyFcn=if exist('tl_reset_reviewflag','file')==2,tl_reset_reviewflag(gcbh);end  DeleteFcn=if exist('delete_tlblock','file')==2,delete_tlblock(gcbh);end  NameChangeFcn=if exist('rename_tlblock','file')==2,rename_tlblock(gcbh);end  OpenFcn=if exist('tl_open_blockdlg','file')==2,tl_open_blockdlg(gcbh);else,open_system(gcbh,'parameter');end
  Switch2 : Switch  Criteria=u2 > Threshold
      settings: CopyFcn=if exist('tl_reset_reviewflag','file')==2,tl_reset_reviewflag(gcbh);end  DeleteFcn=if exist('delete_tlblock','file')==2,delete_tlblock(gcbh);end  NameChangeFcn=if exist('rename_tlblock','file')==2,rename_tlblock(gcbh);end  OpenFcn=if exist('tl_open_blockdlg','file')==2,tl_open_blockdlg(gcbh);else,open_system(gcbh,'parameter');end
  TimeGap : Constant  Value=TimeGap
      settings: CopyFcn=if exist('tl_reset_reviewflag','file')==2,tl_reset_reviewflag(gcbh);end  DeleteFcn=if exist('delete_tlblock','file')==2,delete_tlblock(gcbh);end  NameChangeFcn=if exist('rename_tlblock','file')==2,rename_tlblock(gcbh);end  OpenFcn=if exist('tl_open_blockdlg','file')==2,tl_open_blockdlg(gcbh);else,open_system(gcbh,'parameter');end
  max : MinMax  Function=max  Inputs=2
      settings: CopyFcn=if exist('tl_reset_reviewflag','file')==2,tl_reset_reviewflag(gcbh);end  DeleteFcn=if exist('delete_tlblock','file')==2,delete_tlblock(gcbh);end  NameChangeFcn=if exist('rename_tlblock','file')==2,rename_tlblock(gcbh);end  OpenFcn=if exist('tl_open_blockdlg','file')==2,tl_open_blockdlg(gcbh);else,open_system(gcbh,'parameter');end
  desired_velocity : Outport
  acceleration_parameter : Outport  Port=2
  wires:
  velocity/1 -> max/2
  Divide1/1 -> Sub2/2, Sub1/2
  StandstillDistance/1 -> Sub/2
  pre_distance/1 -> Sub/1
  Sub/1 -> Divide/1
  NoSpeed/1 -> Switch/3
  Divide/1 -> Sub1/1  "Actual Time Gap"
  Sub1/1 -> Switch/2, Switch2/2, Sub2/1
  Sub2/1 -> Switch1/2
  MaxSpeed/1 -> Switch1/1
  pre_velocity/1 -> Switch1/3
  Switch1/1 -> Switch/1
  Switch/1 -> desired_velocity/1
  ComfortAccelerationParameter/1 -> Switch2/1
  Switch2/1 -> acceleration_parameter/1
  FullAcceleartion/1 -> Switch2/3
  StepTimeCoefficient/1 -> Divide1/2
  TimeGap/1 -> Divide1/1
  Epsilon/1 -> max/1
  max/1 -> Divide/2

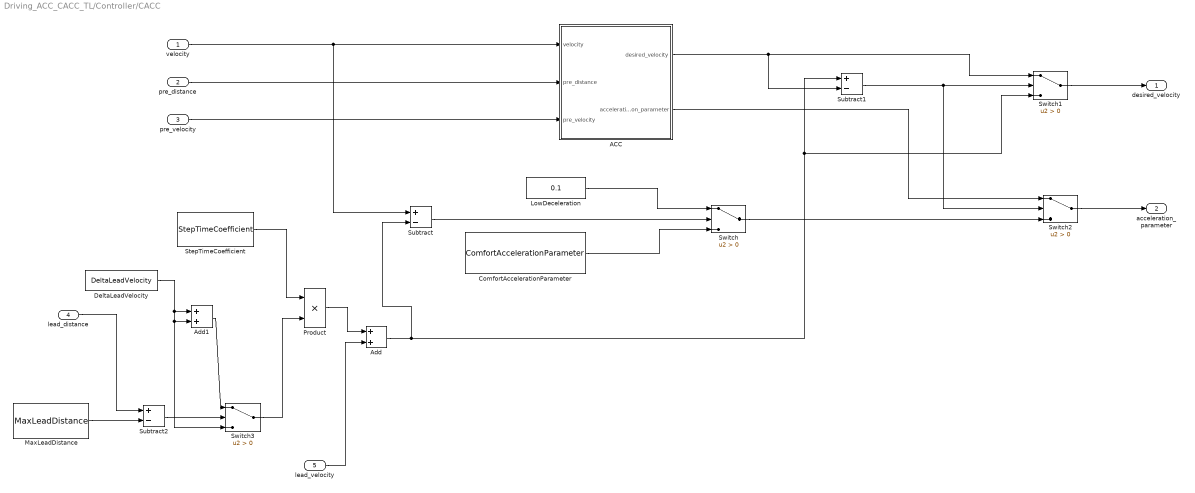
== system Driving_ACC_CACC_TL/Controller/CACC ==
  velocity : Inport
  pre_distance : Inport  Port=2
  pre_velocity : Inport  Port=3
  lead_distance : Inport  Port=4
  lead_velocity : Inport  Port=5
  ACC : Subsystem
  Add : Sum
      settings: CopyFcn=if exist('tl_reset_reviewflag','file')==2,tl_reset_reviewflag(gcbh);end  DeleteFcn=if exist('delete_tlblock','file')==2,delete_tlblock(gcbh);end  NameChangeFcn=if exist('rename_tlblock','file')==2,rename_tlblock(gcbh);end  OpenFcn=if exist('tl_open_blockdlg','file')==2,tl_open_blockdlg(gcbh);else,open_system(gcbh,'parameter');end
  Add1 : Sum
      settings: CopyFcn=if exist('tl_reset_reviewflag','file')==2,tl_reset_reviewflag(gcbh);end  DeleteFcn=if exist('delete_tlblock','file')==2,delete_tlblock(gcbh);end  NameChangeFcn=if exist('rename_tlblock','file')==2,rename_tlblock(gcbh);end  OpenFcn=if exist('tl_open_blockdlg','file')==2,tl_open_blockdlg(gcbh);else,open_system(gcbh,'parameter');end
  ComfortAccelerationParameter : Constant  Value=ComfortAccelerationParameter
      settings: CopyFcn=if exist('tl_reset_reviewflag','file')==2,tl_reset_reviewflag(gcbh);end  DeleteFcn=if exist('delete_tlblock','file')==2,delete_tlblock(gcbh);end  NameChangeFcn=if exist('rename_tlblock','file')==2,rename_tlblock(gcbh);end  OpenFcn=if exist('tl_open_blockdlg','file')==2,tl_open_blockdlg(gcbh);else,open_system(gcbh,'parameter');end
  DeltaLeadVelocity : Constant  Value=DeltaLeadVelocity
      settings: CopyFcn=if exist('tl_reset_reviewflag','file')==2,tl_reset_reviewflag(gcbh);end  DeleteFcn=if exist('delete_tlblock','file')==2,delete_tlblock(gcbh);end  NameChangeFcn=if exist('rename_tlblock','file')==2,rename_tlblock(gcbh);end  OpenFcn=if exist('tl_open_blockdlg','file')==2,tl_open_blockdlg(gcbh);else,open_system(gcbh,'parameter');end
  LowDeceleration : Constant  Value=0.1
      settings: CopyFcn=if exist('tl_reset_reviewflag','file')==2,tl_reset_reviewflag(gcbh);end  DeleteFcn=if exist('delete_tlblock','file')==2,delete_tlblock(gcbh);end  NameChangeFcn=if exist('rename_tlblock','file')==2,rename_tlblock(gcbh);end  OpenFcn=if exist('tl_open_blockdlg','file')==2,tl_open_blockdlg(gcbh);else,open_system(gcbh,'parameter');end
  MaxLeadDistance : Constant  Value=MaxLeadDistance
      settings: CopyFcn=if exist('tl_reset_reviewflag','file')==2,tl_reset_reviewflag(gcbh);end  DeleteFcn=if exist('delete_tlblock','file')==2,delete_tlblock(gcbh);end  NameChangeFcn=if exist('rename_tlblock','file')==2,rename_tlblock(gcbh);end  OpenFcn=if exist('tl_open_blockdlg','file')==2,tl_open_blockdlg(gcbh);else,open_system(gcbh,'parameter');end
  Product : Product
      settings: CopyFcn=if exist('tl_reset_reviewflag','file')==2,tl_reset_reviewflag(gcbh);end  DeleteFcn=if exist('delete_tlblock','file')==2,delete_tlblock(gcbh);end  NameChangeFcn=if exist('rename_tlblock','file')==2,rename_tlblock(gcbh);end  OpenFcn=if exist('tl_open_blockdlg','file')==2,tl_open_blockdlg(gcbh);else,open_system(gcbh,'parameter');end
  StepTimeCoefficient : Constant  Value=StepTimeCoefficient
      settings: CopyFcn=if exist('tl_reset_reviewflag','file')==2,tl_reset_reviewflag(gcbh);end  DeleteFcn=if exist('delete_tlblock','file')==2,delete_tlblock(gcbh);end  NameChangeFcn=if exist('rename_tlblock','file')==2,rename_tlblock(gcbh);end  OpenFcn=if exist('tl_open_blockdlg','file')==2,tl_open_blockdlg(gcbh);else,open_system(gcbh,'parameter');end
  Subtract : Sum  Inputs=+-
      settings: CopyFcn=if exist('tl_reset_reviewflag','file')==2,tl_reset_reviewflag(gcbh);end  DeleteFcn=if exist('delete_tlblock','file')==2,delete_tlblock(gcbh);end  NameChangeFcn=if exist('rename_tlblock','file')==2,rename_tlblock(gcbh);end  OpenFcn=if exist('tl_open_blockdlg','file')==2,tl_open_blockdlg(gcbh);else,open_system(gcbh,'parameter');end
  Subtract1 : Sum  Inputs=+-
      settings: CopyFcn=if exist('tl_reset_reviewflag','file')==2,tl_reset_reviewflag(gcbh);end  DeleteFcn=if exist('delete_tlblock','file')==2,delete_tlblock(gcbh);end  NameChangeFcn=if exist('rename_tlblock','file')==2,rename_tlblock(gcbh);end  OpenFcn=if exist('tl_open_blockdlg','file')==2,tl_open_blockdlg(gcbh);else,open_system(gcbh,'parameter');end
  Subtract2 : Sum  Inputs=+-
      settings: CopyFcn=if exist('tl_reset_reviewflag','file')==2,tl_reset_reviewflag(gcbh);end  DeleteFcn=if exist('delete_tlblock','file')==2,delete_tlblock(gcbh);end  NameChangeFcn=if exist('rename_tlblock','file')==2,rename_tlblock(gcbh);end  OpenFcn=if exist('tl_open_blockdlg','file')==2,tl_open_blockdlg(gcbh);else,open_system(gcbh,'parameter');end
  Switch{,1..3} (4 alike) : Switch  Criteria=u2 > Threshold
      settings: CopyFcn=if exist('tl_reset_reviewflag','file')==2,tl_reset_reviewflag(gcbh);end  DeleteFcn=if exist('delete_tlblock','file')==2,delete_tlblock(gcbh);end  NameChangeFcn=if exist('rename_tlblock','file')==2,rename_tlblock(gcbh);end  OpenFcn=if exist('tl_open_blockdlg','file')==2,tl_open_blockdlg(gcbh);else,open_system(gcbh,'parameter');end
  desired_velocity : Outport
  acceleration_parameter : Outport  Port=2
  wires:
  velocity/1 -> Subtract/1, ACC/1(velocity)
  pre_distance/1 -> ACC/2(pre_distance)
  pre_velocity/1 -> ACC/3(pre_velocity)
  ACC/1(desired_velocity) -> Switch1/1, Subtract1/2
  ACC/2(acceleration_parameter) -> Switch2/1
  lead_velocity/1 -> Add/2
  StepTimeCoefficient/1 -> Product/1
  Product/1 -> Add/1
  Subtract/1 -> Switch/2
  LowDeceleration/1 -> Switch/1
  ComfortAccelerationParameter/1 -> Switch/3
  Switch1/1 -> desired_velocity/1
  Subtract1/1 -> Switch2/2, Switch1/2
  Switch2/1 -> acceleration_parameter/1
  Switch/1 -> Switch2/3
  lead_distance/1 -> Subtract2/1
  MaxLeadDistance/1 -> Subtract2/2
  Add/1 -> Switch1/3, Subtract1/1, Subtract/2
  Switch3/1 -> Product/2
  Subtract2/1 -> Switch3/2
  DeltaLeadVelocity/1 -> Add1/1, Switch3/3, Add1/2
  Add1/1 -> Switch3/1
